simulink model "anubis_deadband3Dof"  (R2024b)
settings: Solver=FixedStepAuto  StartTime=0.0  StopTime=360  FixedStep=.01  RelTol=1e-3
settings Model: Creator=jpajh  LastModifiedBy=djpbj
settings OptimizationCC: OptimizeBlockIOStorage=off  OptimizeDataStoreBuffers=off  BusAssignmentInplaceUpdate=off
settings DebuggingCC: SFUnexpectedBacktrackingDiag=warning  SFNoUnconditionalDefaultTransitionDiag=warning
settings RTWCC: GenCodeOnly=on  GenerateReport=on  BuildConfiguration=Debug  LaunchReport=on
settings CodeAppCC: ForceParamTrailComments=on  MATLABSourceComments=on  EnableCustomComments=on
settings GRTTargetCC: CombineSignalStateStructs=on  SupportVariableSizeSignals=on  MultiInstanceErrorCode=Warning

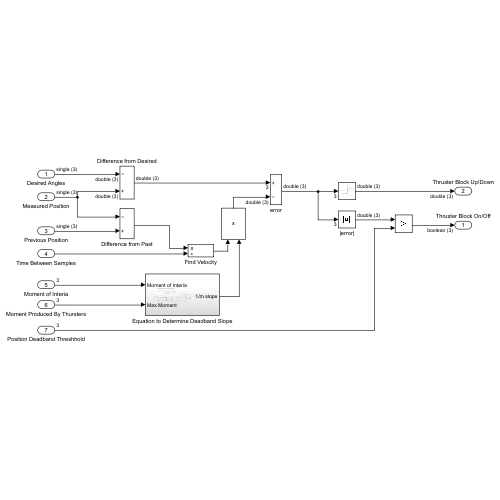
[thumbnail: Simulink's stored preview of the top-level diagram]
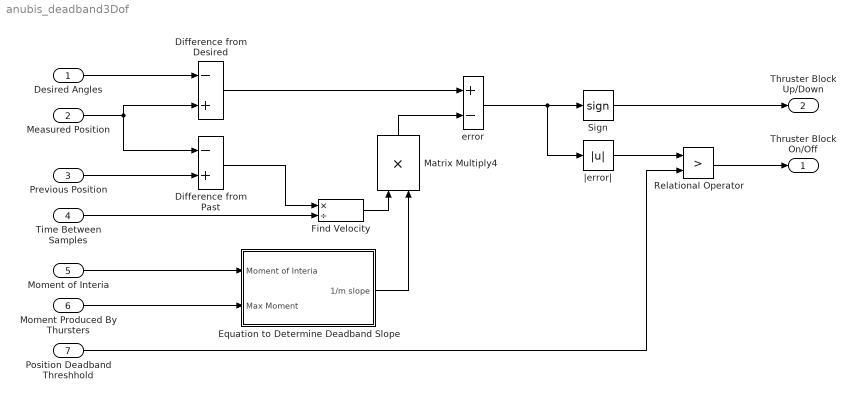
== system anubis_deadband3Dof ==
  Desired Angles : Inport  OutDataTypeStr=single  Unit=deg  PortDimensions=3
  Measured Position : Inport  Port=2  OutDataTypeStr=single  Unit=deg  PortDimensions=3
  Previous Position : Inport  Port=3  OutDataTypeStr=single  Unit=deg  PortDimensions=3
  Time Between Samples : Inport  Port=4  Unit=sec  PortDimensions=1
  Moment of Interia : Inport  Port=5  Unit=kg*m^2  PortDimensions=3
  Moment Produced By Thursters : Inport  Port=6  Unit=N*m  PortDimensions=3
  Position Deadband Threshhold : Inport  Port=7  Unit=deg  PortDimensions=3
  Difference from Desired : Sum  Inputs=-+
  Difference from Past : Sum  Inputs=-+
  Equation to Determine Deadband Slope : Subsystem
  Find Velocity : Product  Inputs=*/
  Matrix Multiply4 : Product
  Relational Operator : RelationalOperator  Operator=>  OutDataTypeStr=boolean  RndMeth=Simplest  InputSameDT=off
  Sign : Signum
  error : Sum  Inputs=+-
  |error| : Abs  SaturateOnIntegerOverflow=off
  Thruster Block On/Off : Outport  OutDataTypeStr=boolean  PortDimensions=3
  Thruster Block Up/Down : Outport  Port=2  OutDataTypeStr=double  PortDimensions=3
  wires:
  |error|/1 -> Relational Operator/1
  Sign/1 -> Thruster Block Up/Down/1
  Desired Angles/1 -> Difference from Desired/1
  Relational Operator/1 -> Thruster Block On/Off/1
  Difference from Desired/1 -> error/1
  error/1 -> Sign/1, |error|/1
  Position Deadband Threshhold/1 -> Relational Operator/2
  Moment of Interia/1 -> Equation to Determine Deadband Slope/1(Moment of Interia)
  Moment Produced By Thursters/1 -> Equation to Determine Deadband Slope/2(Max Moment)
  Matrix Multiply4/1 -> error/2
  Measured Position/1 -> Difference from Past/1, Difference from Desired/2
  Time Between Samples/1 -> Find Velocity/2
  Previous Position/1 -> Difference from Past/2
  Difference from Past/1 -> Find Velocity/1
  Find Velocity/1 -> Matrix Multiply4/1
  Equation to Determine Deadband Slope/1(1/m slope) -> Matrix Multiply4/2

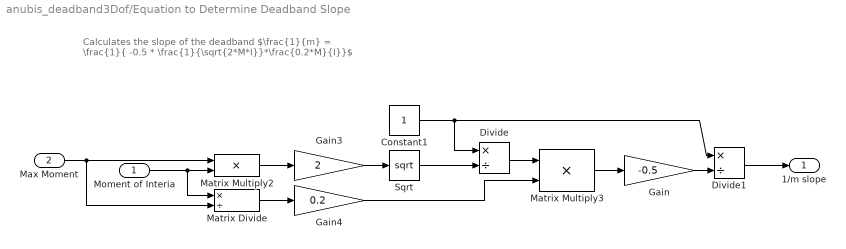
== system anubis_deadband3Dof/Equation to Determine Deadband Slope ==
  note: Calculates the slope of the deadband
      | $\frac{1}{m} = \frac{1}{ -0.5 * \frac{1}{\sqrt{2*M*I}}*\frac{0.2*M}{I}}$
  Moment of Interia : Inport
  Max Moment : Inport  Port=2
  Constant1 : Constant
  Divide : Product  Inputs=*/
  Divide1 : Product  Inputs=*/
  Gain : Gain  Gain=-0.5
  Gain3 : Gain  Gain=2
  Gain4 : Gain  Gain=0.2
  Matrix Divide : Product  Inputs=*/
  Matrix Multiply2 : Product
  Matrix Multiply3 : Product
  Sqrt : Sqrt
  1/m slope : Outport
  wires:
  Matrix Divide/1 -> Gain4/1
  Divide1/1 -> 1/m slope/1
  Gain/1 -> Divide1/2
  Constant1/1 -> Divide/1, Divide1/1
  Matrix Multiply3/1 -> Gain/1
  Sqrt/1 -> Divide/2
  Divide/1 -> Matrix Multiply3/1
  Matrix Multiply2/1 -> Gain3/1
  Gain4/1 -> Matrix Multiply3/2
  Gain3/1 -> Sqrt/1
  Max Moment/1 -> Matrix Multiply2/1, Matrix Divide/2
  Moment of Interia/1 -> Matrix Divide/1, Matrix Multiply2/2
